simulink model "goertzel"  (R2020a)
settings: Solver=FixedStepAuto  StartTime=0.0  StopTime=3  FixedStep=1/16000  RelTol=1e-3
libraries: audiosources x1, dspvision x1
settings Model: Creator=gonze  LastModifiedBy=ricar

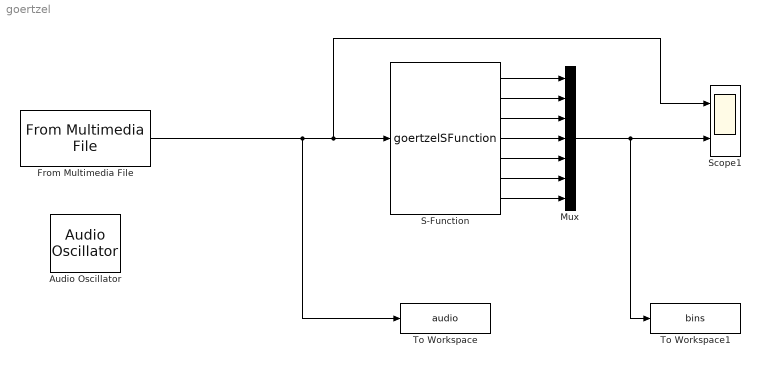
== system goertzel ==
  Audio Oscillator : audiosources/Audio Oscillator  FrequencyPort=off  Frequency=700  AmplitudePort=off  Amplitude=1  DCOffsetPort=off  PhaseOffset=0  DCOffset=0  WidthPort=off  Width=1  DutyCyclePort=off  DutyCycle=0.5  SampsPerFrame=1  Fs=16000  OutputDataType=double  SimulateUsing=Code generation
      settings: SourceProductBaseCode=AU  SignalType=sine
  From Multimedia File : dspvision/From Multimedia File  inputFilename=C:\Users\ricar\Desktop\Lab-DSP\lab4dsp_G6_Graves_Mardones\labC\sources\s-function_goertzel\dtmfSequence_16_16.wav  readRange=[1 Inf]  loop=on  numPlays=1  outputStreams=Audio only  videoDataType=single  audioDataType=double  inheritSampleTime=on  userDefinedSampleTime=1/30  noAudioOutput=off  isIntensityVideo=off  fourcc=RGB  colorVideoFormat=Separate color signals  outputEOF=off  dataOrg=Column-major  audioFrameSize=1  computeAudioFrameSize=off  outSamplingMode=Sample based
  Mux : Mux  Inputs=7
  S-Function : S-Function  FunctionName=goertzelSFunction  SFunctionDeploymentMode=off  EnableBusSupport=off
  Scope1 : Scope  NumInputPorts=2
  To Workspace : ToWorkspace  VariableName=audio  SampleTime=-1
      settings: Save2DSignal=2-D array (concatenate along first dimension)
  To Workspace1 : ToWorkspace  VariableName=bins  SampleTime=-1
      settings: Save2DSignal=2-D array (concatenate along first dimension)
  wires:
  Mux/1 -> To Workspace1/1, Scope1/2
  From Multimedia File/1 -> Scope1/1, S-Function/1, To Workspace/1
  S-Function/4 -> Mux/4
  S-Function/3 -> Mux/3
  S-Function/2 -> Mux/2
  S-Function/1 -> Mux/1
  S-Function/5 -> Mux/5
  S-Function/6 -> Mux/6
  S-Function/7 -> Mux/7
